simulink model "Power_Grid_Fault_Analysis_"  (R2019b)
settings: Solver=FixedStepAuto  StartTime=0.0  StopTime=0.2  RelTol=1e-3
InitFcn:
  | basekV = 23;
  | baseMVA = 100;
  | 
  | % base impedance
  | baseZ = (basekV)^2/baseMVA;
  | 
  | % nominal frequency
  | freq = 50;
libraries: powerlib x64, powerlib_meascontrol x17
(part 4 of 4)

== system Power_Grid_Fault_Analysis_/For Zone 2/If Action Subsystem1 ==
  Input : Inport
  Input1 : Inport  Port=2
  Input2 : Inport  Port=3
  Action Port : ActionPort  ActionPortLabel=elseif(u5 <= u1 & u1 <=u4 & u5 <= u3 & u3 <= u4 & u2 < u6)
  Out1 : Outport
  Out2 : Outport  Port=2
  Out3 : Outport  Port=3
  wires:
  Input/1 -> Out1/1
  Input1/1 -> Out2/1
  Input2/1 -> Out3/1

== system Power_Grid_Fault_Analysis_/For Zone 2/If Action Subsystem2 ==
  Input : Inport
  Input1 : Inport  Port=2
  Input2 : Inport  Port=3
  Action Port : ActionPort  ActionPortLabel=if(u5 <= u1 & u1 <=u4 & u5 <= u2 & u2 <=u4 & u3< u6)
  Out1 : Outport
  Out2 : Outport  Port=2
  Out3 : Outport  Port=3
  wires:
  Input/1 -> Out1/1
  Input1/1 -> Out2/1
  Input2/1 -> Out3/1

== system Power_Grid_Fault_Analysis_/For Zone 2/If Action Subsystem3 ==
  Input : Inport
  Input1 : Inport  Port=2
  Input2 : Inport  Port=3
  Action Port : ActionPort  ActionPortLabel=elseif(45 <= u3 & u3 <=u4 & u1 <= u7 & u2 <= u7)
  Out1 : Outport
  Out2 : Outport  Port=2
  Out3 : Outport  Port=3
  wires:
  Input/1 -> Out1/1
  Input1/1 -> Out2/1
  Input2/1 -> Out3/1

== system Power_Grid_Fault_Analysis_/For Zone 2/If Action Subsystem4 ==
  Input : Inport
  Input1 : Inport  Port=2
  Input2 : Inport  Port=3
  Action Port : ActionPort  ActionPortLabel="if(u1 >u5 & u2<u5 &  u3<u5)"
  Out1 : Outport
  Out2 : Outport  Port=2
  Out3 : Outport  Port=3
  wires:
  Input/1 -> Out1/1
  Input1/1 -> Out2/1
  Input2/1 -> Out3/1

== system Power_Grid_Fault_Analysis_/For Zone 2/If Action Subsystem5 ==
  Input : Inport
  Input1 : Inport  Port=2
  Input2 : Inport  Port=3
  Action Port : ActionPort  ActionPortLabel="elseif(u1 <u5 & u2>u5 &  u3<u5)"
  Out1 : Outport
  Out2 : Outport  Port=2
  Out3 : Outport  Port=3
  wires:
  Input/1 -> Out1/1
  Input1/1 -> Out2/1
  Input2/1 -> Out3/1

== system Power_Grid_Fault_Analysis_/For Zone 2/If Action Subsystem6 ==
  Input : Inport
  Input1 : Inport  Port=2
  Input2 : Inport  Port=3
  Action Port : ActionPort  ActionPortLabel="if(0<u1 & u1 < u4  &  u2 < u4 &  u3 <u4)"
  Out1 : Outport
  Out2 : Outport  Port=2
  Out3 : Outport  Port=3
  wires:
  Input/1 -> Out1/1
  Input1/1 -> Out2/1
  Input2/1 -> Out3/1

== system Power_Grid_Fault_Analysis_/For Zone 2/Subsystem1 ==
  In1 : Inport
  In2 : Inport  Port=2
  Display2 : Display
      settings: Decimation=2
  Divide4 : Product  Inputs=**  SaturateOnIntegerOverflow=on  RndMeth=Zero
  Output : Outport
  wires:
  Divide4/1 -> Display2/1, Output/1
  In1/1 -> Divide4/1
  In2/1 -> Divide4/2

== system Power_Grid_Fault_Analysis_/For Zone 2/Subsystem2 ==
  In1 : Inport
  In2 : Inport  Port=2
  Display2 : Display
      settings: Decimation=2
  Divide4 : Product  Inputs=**  SaturateOnIntegerOverflow=on  RndMeth=Zero
  Output : Outport
  wires:
  In2/1 -> Divide4/2
  In1/1 -> Divide4/1
  Divide4/1 -> Output/1, Display2/1

== system Power_Grid_Fault_Analysis_/For Zone 2/Subsystem3 ==
  In1 : Inport
  In2 : Inport  Port=2
  Display2 : Display
      settings: Decimation=2
  Divide4 : Product  Inputs=**  SaturateOnIntegerOverflow=on  RndMeth=Zero
  Output : Outport
  wires:
  In2/1 -> Divide4/2
  In1/1 -> Divide4/1
  Divide4/1 -> Output/1, Display2/1

== system Power_Grid_Fault_Analysis_/For Zone 2/Subsystem4 ==
  In1 : Inport
  In2 : Inport  Port=2
  Display2 : Display
      settings: Decimation=2
  Divide4 : Product  Inputs=**  SaturateOnIntegerOverflow=on  RndMeth=Zero
  Output : Outport
  wires:
  Divide4/1 -> Display2/1, Output/1
  In1/1 -> Divide4/1
  In2/1 -> Divide4/2

== system Power_Grid_Fault_Analysis_/For Zone 2/Subsystem5 ==
  In1 : Inport
  In2 : Inport  Port=2
  Display2 : Display
      settings: Decimation=2
  Divide4 : Product  Inputs=**  SaturateOnIntegerOverflow=on  RndMeth=Zero
  Output : Outport
  wires:
  In2/1 -> Divide4/2
  In1/1 -> Divide4/1
  Divide4/1 -> Output/1, Display2/1

== system Power_Grid_Fault_Analysis_/For Zone 2/Subsystem6 ==
  In1 : Inport
  In2 : Inport  Port=2
  Display2 : Display
      settings: Decimation=2
  Divide4 : Product  Inputs=**  SaturateOnIntegerOverflow=on  RndMeth=Zero
  Output : Outport
  wires:
  Divide4/1 -> Display2/1, Output/1
  In1/1 -> Divide4/1
  In2/1 -> Divide4/2

== system Power_Grid_Fault_Analysis_/For Zone 2/Subsystem7 ==
  In1 : Inport
  In2 : Inport  Port=2
  Display2 : Display
      settings: Decimation=2
  Divide4 : Product  Inputs=**  SaturateOnIntegerOverflow=on  RndMeth=Zero
  Output : Outport
  wires:
  In2/1 -> Divide4/2
  In1/1 -> Divide4/1
  Divide4/1 -> Output/1, Display2/1

== system Power_Grid_Fault_Analysis_/For Zone 3/If Action Subsystem ==
  Input : Inport
  Input1 : Inport  Port=2
  Input2 : Inport  Port=3
  Action Port : ActionPort  ActionPortLabel=if(u5 <= u2 & u2 <=u4 & u5 <= u3 & u3 <=u4 & u1 < u6)
  Out1 : Outport
  Out2 : Outport  Port=2
  Out3 : Outport  Port=3
  wires:
  Input/1 -> Out1/1
  Input1/1 -> Out2/1
  Input2/1 -> Out3/1

== system Power_Grid_Fault_Analysis_/For Zone 3/If Action Subsystem1 ==
  Input : Inport
  Input1 : Inport  Port=2
  Input2 : Inport  Port=3
  Action Port : ActionPort  ActionPortLabel=elseif(u5 <= u1 & u1 <=u4 & u5 <= u3 & u3 <= u4 & u2 < u6)
  Out1 : Outport
  Out2 : Outport  Port=2
  Out3 : Outport  Port=3
  wires:
  Input/1 -> Out1/1
  Input1/1 -> Out2/1
  Input2/1 -> Out3/1

== system Power_Grid_Fault_Analysis_/For Zone 3/If Action Subsystem2 ==
  Input : Inport
  Input1 : Inport  Port=2
  Input2 : Inport  Port=3
  Action Port : ActionPort  ActionPortLabel=if(u5 <= u1 & u1 <=u4 & u5 <= u2 & u2 <=u4 & u3< u6)
  Out1 : Outport
  Out2 : Outport  Port=2
  Out3 : Outport  Port=3
  wires:
  Input/1 -> Out1/1
  Input1/1 -> Out2/1
  Input2/1 -> Out3/1

== system Power_Grid_Fault_Analysis_/For Zone 3/If Action Subsystem3 ==
  Input : Inport
  Input1 : Inport  Port=2
  Input2 : Inport  Port=3
  Action Port : ActionPort  ActionPortLabel=elseif(15<= u3 & u3 <=u4 & u1 <= u7 & u2 <= u7)
  Out1 : Outport
  Out2 : Outport  Port=2
  Out3 : Outport  Port=3
  wires:
  Input/1 -> Out1/1
  Input1/1 -> Out2/1
  Input2/1 -> Out3/1

== system Power_Grid_Fault_Analysis_/For Zone 3/If Action Subsystem4 ==
  Input : Inport
  Input1 : Inport  Port=2
  Input2 : Inport  Port=3
  Action Port : ActionPort  ActionPortLabel="if(u1 >u5 & u2<u5 &  u3<u5)"
  Out1 : Outport
  Out2 : Outport  Port=2
  Out3 : Outport  Port=3
  wires:
  Input/1 -> Out1/1
  Input1/1 -> Out2/1
  Input2/1 -> Out3/1

== system Power_Grid_Fault_Analysis_/For Zone 3/If Action Subsystem5 ==
  Input : Inport
  Input1 : Inport  Port=2
  Input2 : Inport  Port=3
  Action Port : ActionPort  ActionPortLabel="elseif(u1 <u5 & u2>u5 &  u3<u5)"
  Out1 : Outport
  Out2 : Outport  Port=2
  Out3 : Outport  Port=3
  wires:
  Input/1 -> Out1/1
  Input1/1 -> Out2/1
  Input2/1 -> Out3/1

== system Power_Grid_Fault_Analysis_/For Zone 3/If Action Subsystem6 ==
  Input : Inport
  Input1 : Inport  Port=2
  Input2 : Inport  Port=3
  Action Port : ActionPort  ActionPortLabel="if(0<u1 & u1 < u4  &  u2 < u4 &  u3 <u4)"
  Out1 : Outport
  Out2 : Outport  Port=2
  Out3 : Outport  Port=3
  wires:
  Input/1 -> Out1/1
  Input1/1 -> Out2/1
  Input2/1 -> Out3/1

== system Power_Grid_Fault_Analysis_/For Zone 3/Subsystem1 ==
  In1 : Inport
  In2 : Inport  Port=2
  Display2 : Display
      settings: Decimation=2
  Divide4 : Product  Inputs=**  SaturateOnIntegerOverflow=on  RndMeth=Zero
  Output : Outport
  wires:
  Divide4/1 -> Display2/1, Output/1
  In1/1 -> Divide4/1
  In2/1 -> Divide4/2

== system Power_Grid_Fault_Analysis_/For Zone 3/Subsystem2 ==
  In1 : Inport
  In2 : Inport  Port=2
  Display2 : Display
      settings: Decimation=2
  Divide4 : Product  Inputs=**  SaturateOnIntegerOverflow=on  RndMeth=Zero
  Output : Outport
  wires:
  In2/1 -> Divide4/2
  In1/1 -> Divide4/1
  Divide4/1 -> Output/1, Display2/1

== system Power_Grid_Fault_Analysis_/For Zone 3/Subsystem3 ==
  In1 : Inport
  In2 : Inport  Port=2
  Display2 : Display
      settings: Decimation=2
  Divide4 : Product  Inputs=**  SaturateOnIntegerOverflow=on  RndMeth=Zero
  Output : Outport
  wires:
  In2/1 -> Divide4/2
  In1/1 -> Divide4/1
  Divide4/1 -> Output/1, Display2/1

== system Power_Grid_Fault_Analysis_/For Zone 3/Subsystem4 ==
  In1 : Inport
  In2 : Inport  Port=2
  Display2 : Display
      settings: Decimation=2
  Divide4 : Product  Inputs=**  SaturateOnIntegerOverflow=on  RndMeth=Zero
  Output : Outport
  wires:
  Divide4/1 -> Display2/1, Output/1
  In1/1 -> Divide4/1
  In2/1 -> Divide4/2

== system Power_Grid_Fault_Analysis_/For Zone 3/Subsystem5 ==
  In1 : Inport
  In2 : Inport  Port=2
  Display2 : Display
      settings: Decimation=2
  Divide4 : Product  Inputs=**  SaturateOnIntegerOverflow=on  RndMeth=Zero
  Output : Outport
  wires:
  In2/1 -> Divide4/2
  In1/1 -> Divide4/1
  Divide4/1 -> Output/1, Display2/1

== system Power_Grid_Fault_Analysis_/For Zone 3/Subsystem6 ==
  In1 : Inport
  In2 : Inport  Port=2
  Display2 : Display
      settings: Decimation=2
  Divide4 : Product  Inputs=**  SaturateOnIntegerOverflow=on  RndMeth=Zero
  Output : Outport
  wires:
  Divide4/1 -> Display2/1, Output/1
  In1/1 -> Divide4/1
  In2/1 -> Divide4/2

== system Power_Grid_Fault_Analysis_/For Zone 3/Subsystem7 ==
  In1 : Inport
  In2 : Inport  Port=2
  Display2 : Display
      settings: Decimation=2
  Divide4 : Product  Inputs=**  SaturateOnIntegerOverflow=on  RndMeth=Zero
  Output : Outport
  wires:
  In2/1 -> Divide4/2
  In1/1 -> Divide4/1
  Divide4/1 -> Output/1, Display2/1

== system Power_Grid_Fault_Analysis_/For Zone 4/If Action Subsystem ==
  Input : Inport
  Input1 : Inport  Port=2
  Input2 : Inport  Port=3
  Action Port : ActionPort  ActionPortLabel=if(u5 <= u2 & u2 <=u4 & u5 <= u3 & u3 <=u4 & u1 < u6)
  Out1 : Outport
  Out2 : Outport  Port=2
  Out3 : Outport  Port=3
  wires:
  Input/1 -> Out1/1
  Input1/1 -> Out2/1
  Input2/1 -> Out3/1

== system Power_Grid_Fault_Analysis_/For Zone 4/If Action Subsystem1 ==
  Input : Inport
  Input1 : Inport  Port=2
  Input2 : Inport  Port=3
  Action Port : ActionPort  ActionPortLabel=elseif(u5 <= u1 & u1 <=u4 & u5 <= u3 & u3 <= u4 & u2 < u6)
  Out1 : Outport
  Out2 : Outport  Port=2
  Out3 : Outport  Port=3
  wires:
  Input/1 -> Out1/1
  Input1/1 -> Out2/1
  Input2/1 -> Out3/1

== system Power_Grid_Fault_Analysis_/For Zone 4/If Action Subsystem2 ==
  Input : Inport
  Input1 : Inport  Port=2
  Input2 : Inport  Port=3
  Action Port : ActionPort  ActionPortLabel=if(u5 <= u1 & u1 <=u4 & u5 <= u2 & u2 <=u4 & u3< u6)
  Out1 : Outport
  Out2 : Outport  Port=2
  Out3 : Outport  Port=3
  wires:
  Input/1 -> Out1/1
  Input1/1 -> Out2/1
  Input2/1 -> Out3/1

== system Power_Grid_Fault_Analysis_/For Zone 4/If Action Subsystem3 ==
  Input : Inport
  Input1 : Inport  Port=2
  Input2 : Inport  Port=3
  Action Port : ActionPort  ActionPortLabel=elseif(120 <= u3 & u3 <=u4 & u1 <= u7 & u2 <= u7)
  Out1 : Outport
  Out2 : Outport  Port=2
  Out3 : Outport  Port=3
  wires:
  Input/1 -> Out1/1
  Input1/1 -> Out2/1
  Input2/1 -> Out3/1

== system Power_Grid_Fault_Analysis_/For Zone 4/If Action Subsystem4 ==
  Input : Inport
  Input1 : Inport  Port=2
  Input2 : Inport  Port=3
  Action Port : ActionPort  ActionPortLabel="if(u1 >u5 & u2<u5 &  u3<u5)"
  Out1 : Outport
  Out2 : Outport  Port=2
  Out3 : Outport  Port=3
  wires:
  Input/1 -> Out1/1
  Input1/1 -> Out2/1
  Input2/1 -> Out3/1

== system Power_Grid_Fault_Analysis_/For Zone 4/If Action Subsystem5 ==
  Input : Inport
  Input1 : Inport  Port=2
  Input2 : Inport  Port=3
  Action Port : ActionPort  ActionPortLabel="elseif(u1 <u5 & u2>u5 &  u3<u5)"
  Out1 : Outport
  Out2 : Outport  Port=2
  Out3 : Outport  Port=3
  wires:
  Input/1 -> Out1/1
  Input1/1 -> Out2/1
  Input2/1 -> Out3/1

== system Power_Grid_Fault_Analysis_/For Zone 4/If Action Subsystem6 ==
  Input : Inport
  Input1 : Inport  Port=2
  Input2 : Inport  Port=3
  Action Port : ActionPort  ActionPortLabel="if(0<u1 & u1 < u4  &  u2 < u4 &  u3 <u4)"
  Out1 : Outport
  Out2 : Outport  Port=2
  Out3 : Outport  Port=3
  wires:
  Input/1 -> Out1/1
  Input1/1 -> Out2/1
  Input2/1 -> Out3/1

== system Power_Grid_Fault_Analysis_/For Zone 4/Subsystem1 ==
  In1 : Inport
  In2 : Inport  Port=2
  Display2 : Display
      settings: Decimation=2
  Divide4 : Product  Inputs=**  SaturateOnIntegerOverflow=on  RndMeth=Zero
  Output : Outport
  wires:
  Divide4/1 -> Display2/1, Output/1
  In1/1 -> Divide4/1
  In2/1 -> Divide4/2

== system Power_Grid_Fault_Analysis_/For Zone 4/Subsystem2 ==
  In1 : Inport
  In2 : Inport  Port=2
  Display2 : Display
      settings: Decimation=2
  Divide4 : Product  Inputs=**  SaturateOnIntegerOverflow=on  RndMeth=Zero
  Output : Outport
  wires:
  In2/1 -> Divide4/2
  In1/1 -> Divide4/1
  Divide4/1 -> Output/1, Display2/1

== system Power_Grid_Fault_Analysis_/For Zone 4/Subsystem3 ==
  In1 : Inport
  In2 : Inport  Port=2
  Display2 : Display
      settings: Decimation=2
  Divide4 : Product  Inputs=**  SaturateOnIntegerOverflow=on  RndMeth=Zero
  Output : Outport
  wires:
  In2/1 -> Divide4/2
  In1/1 -> Divide4/1
  Divide4/1 -> Output/1, Display2/1

== system Power_Grid_Fault_Analysis_/For Zone 4/Subsystem4 ==
  In1 : Inport
  In2 : Inport  Port=2
  Display2 : Display
      settings: Decimation=2
  Divide4 : Product  Inputs=**  SaturateOnIntegerOverflow=on  RndMeth=Zero
  Output : Outport
  wires:
  Divide4/1 -> Display2/1, Output/1
  In1/1 -> Divide4/1
  In2/1 -> Divide4/2

== system Power_Grid_Fault_Analysis_/For Zone 4/Subsystem5 ==
  In1 : Inport
  In2 : Inport  Port=2
  Display2 : Display
      settings: Decimation=2
  Divide4 : Product  Inputs=**  SaturateOnIntegerOverflow=on  RndMeth=Zero
  Output : Outport
  wires:
  In2/1 -> Divide4/2
  In1/1 -> Divide4/1
  Divide4/1 -> Output/1, Display2/1

== system Power_Grid_Fault_Analysis_/For Zone 4/Subsystem6 ==
  In1 : Inport
  In2 : Inport  Port=2
  Display2 : Display
      settings: Decimation=2
  Divide4 : Product  Inputs=**  SaturateOnIntegerOverflow=on  RndMeth=Zero
  Output : Outport
  wires:
  Divide4/1 -> Display2/1, Output/1
  In1/1 -> Divide4/1
  In2/1 -> Divide4/2

== system Power_Grid_Fault_Analysis_/For Zone 4/Subsystem7 ==
  In1 : Inport
  In2 : Inport  Port=2
  Display2 : Display
      settings: Decimation=2
  Divide4 : Product  Inputs=**  SaturateOnIntegerOverflow=on  RndMeth=Zero
  Output : Outport
  wires:
  In2/1 -> Divide4/2
  In1/1 -> Divide4/1
  Divide4/1 -> Output/1, Display2/1

== system Power_Grid_Fault_Analysis_/For Zone 5/If Action Subsystem ==
  Input : Inport
  Input1 : Inport  Port=2
  Input2 : Inport  Port=3
  Action Port : ActionPort  ActionPortLabel=if(u5 <= u2 & u2 <=u4 & u5 <= u3 & u3 <=u4 & u1 < u6)
  Out1 : Outport
  Out2 : Outport  Port=2
  Out3 : Outport  Port=3
  wires:
  Input/1 -> Out1/1
  Input1/1 -> Out2/1
  Input2/1 -> Out3/1

== system Power_Grid_Fault_Analysis_/For Zone 5/If Action Subsystem1 ==
  Input : Inport
  Input1 : Inport  Port=2
  Input2 : Inport  Port=3
  Action Port : ActionPort  ActionPortLabel=elseif(u5 <= u1 & u1 <=u4 & u5 <= u3 & u3 <= u4 & u2 < u6)
  Out1 : Outport
  Out2 : Outport  Port=2
  Out3 : Outport  Port=3
  wires:
  Input/1 -> Out1/1
  Input1/1 -> Out2/1
  Input2/1 -> Out3/1

== system Power_Grid_Fault_Analysis_/For Zone 5/If Action Subsystem2 ==
  Input : Inport
  Input1 : Inport  Port=2
  Input2 : Inport  Port=3
  Action Port : ActionPort  ActionPortLabel=if(u5 <= u1 & u1 <=u4 & u5 <= u2 & u2 <=u4 & u3< u6)
  Out1 : Outport
  Out2 : Outport  Port=2
  Out3 : Outport  Port=3
  wires:
  Input/1 -> Out1/1
  Input1/1 -> Out2/1
  Input2/1 -> Out3/1

== system Power_Grid_Fault_Analysis_/For Zone 5/If Action Subsystem3 ==
  Input : Inport
  Input1 : Inport  Port=2
  Input2 : Inport  Port=3
  Action Port : ActionPort  ActionPortLabel=elseif(50 <= u3 & u3 <=u4 & u1 <= u7 & u2 <= u7)
  Out1 : Outport
  Out2 : Outport  Port=2
  Out3 : Outport  Port=3
  wires:
  Input/1 -> Out1/1
  Input1/1 -> Out2/1
  Input2/1 -> Out3/1

== system Power_Grid_Fault_Analysis_/For Zone 5/If Action Subsystem4 ==
  Input : Inport
  Input1 : Inport  Port=2
  Input2 : Inport  Port=3
  Action Port : ActionPort  ActionPortLabel="if(u1 >u5 & u2<u5 &  u3<u5)"
  Out1 : Outport
  Out2 : Outport  Port=2
  Out3 : Outport  Port=3
  wires:
  Input/1 -> Out1/1
  Input1/1 -> Out2/1
  Input2/1 -> Out3/1

== system Power_Grid_Fault_Analysis_/For Zone 5/If Action Subsystem5 ==
  Input : Inport
  Input1 : Inport  Port=2
  Input2 : Inport  Port=3
  Action Port : ActionPort  ActionPortLabel="elseif(u1 <u5 & u2>u5 &  u3<u5)"
  Out1 : Outport
  Out2 : Outport  Port=2
  Out3 : Outport  Port=3
  wires:
  Input/1 -> Out1/1
  Input1/1 -> Out2/1
  Input2/1 -> Out3/1

== system Power_Grid_Fault_Analysis_/For Zone 5/If Action Subsystem6 ==
  Input : Inport
  Input1 : Inport  Port=2
  Input2 : Inport  Port=3
  Action Port : ActionPort  ActionPortLabel="if(0<u1 & u1 < u4  &  u2 < u4 &  u3 <u4)"
  Out1 : Outport
  Out2 : Outport  Port=2
  Out3 : Outport  Port=3
  wires:
  Input/1 -> Out1/1
  Input1/1 -> Out2/1
  Input2/1 -> Out3/1

== system Power_Grid_Fault_Analysis_/For Zone 5/Subsystem1 ==
  In1 : Inport
  In2 : Inport  Port=2
  Display2 : Display
      settings: Decimation=2
  Divide4 : Product  Inputs=**  SaturateOnIntegerOverflow=on  RndMeth=Zero
  Output : Outport
  wires:
  Divide4/1 -> Display2/1, Output/1
  In1/1 -> Divide4/1
  In2/1 -> Divide4/2

== system Power_Grid_Fault_Analysis_/For Zone 5/Subsystem2 ==
  In1 : Inport
  In2 : Inport  Port=2
  Display2 : Display
      settings: Decimation=2
  Divide4 : Product  Inputs=**  SaturateOnIntegerOverflow=on  RndMeth=Zero
  Output : Outport
  wires:
  In2/1 -> Divide4/2
  In1/1 -> Divide4/1
  Divide4/1 -> Output/1, Display2/1

== system Power_Grid_Fault_Analysis_/For Zone 5/Subsystem3 ==
  In1 : Inport
  In2 : Inport  Port=2
  Display2 : Display
      settings: Decimation=2
  Divide4 : Product  Inputs=**  SaturateOnIntegerOverflow=on  RndMeth=Zero
  Output : Outport
  wires:
  In2/1 -> Divide4/2
  In1/1 -> Divide4/1
  Divide4/1 -> Output/1, Display2/1

== system Power_Grid_Fault_Analysis_/For Zone 5/Subsystem4 ==
  In1 : Inport
  In2 : Inport  Port=2
  Display2 : Display
      settings: Decimation=2
  Divide4 : Product  Inputs=**  SaturateOnIntegerOverflow=on  RndMeth=Zero
  Output : Outport
  wires:
  Divide4/1 -> Display2/1, Output/1
  In1/1 -> Divide4/1
  In2/1 -> Divide4/2

== system Power_Grid_Fault_Analysis_/For Zone 5/Subsystem5 ==
  In1 : Inport
  In2 : Inport  Port=2
  Display2 : Display
      settings: Decimation=2
  Divide4 : Product  Inputs=**  SaturateOnIntegerOverflow=on  RndMeth=Zero
  Output : Outport
  wires:
  In2/1 -> Divide4/2
  In1/1 -> Divide4/1
  Divide4/1 -> Output/1, Display2/1

== system Power_Grid_Fault_Analysis_/For Zone 5/Subsystem6 ==
  In1 : Inport
  In2 : Inport  Port=2
  Display2 : Display
      settings: Decimation=2
  Divide4 : Product  Inputs=**  SaturateOnIntegerOverflow=on  RndMeth=Zero
  Output : Outport
  wires:
  Divide4/1 -> Display2/1, Output/1
  In1/1 -> Divide4/1
  In2/1 -> Divide4/2

== system Power_Grid_Fault_Analysis_/For Zone 5/Subsystem7 ==
  In1 : Inport
  In2 : Inport  Port=2
  Display2 : Display
      settings: Decimation=2
  Divide4 : Product  Inputs=**  SaturateOnIntegerOverflow=on  RndMeth=Zero
  Output : Outport
  wires:
  In2/1 -> Divide4/2
  In1/1 -> Divide4/1
  Divide4/1 -> Output/1, Display2/1

== system Power_Grid_Fault_Analysis_/Relay /AC Time Overcurrent Relay2 ==
  I : Inport
  Clock : Clock
  Irms : powerlib_meascontrol/Measurements/RMS  TrueRMS=on  Freq=Freq  RMSInit=RMSInit  Ts=0
      settings: SourceProductName=Simscape Electrical
  Relational Operator : RelationalOperator  Operator=<=  OutDataTypeStr=boolean  RndMeth=Nearest
  Time Relay Function : MATLAB Function  TreatAsAtomicUnit=on
  C.B : Outport
  OT : Outport  Port=2
  wires:
  Clock/1 -> Relational Operator/1, Time Relay Function/1(clk)
  Irms/1 -> Time Relay Function/2(Irms)
  Time Relay Function/1(TT) -> Relational Operator/2
  Time Relay Function/2(OT) -> OT/1
  Relational Operator/1 -> C.B/1
  I/1 -> Irms/1

== system Power_Grid_Fault_Analysis_/Relay /Output1 ==
  Signal : Inport
  Demux : Demux  Outputs=3
  Scope : Scope  NumInputPorts=3
  wires:
  Demux/3 -> Scope/3
  Demux/1 -> Scope/1
  Demux/2 -> Scope/2
  Signal/1 -> Demux/1

== system Power_Grid_Fault_Analysis_/Relay /Subsystem ==
  In1 : Inport
  Constant : Constant  Value=5
  Data Type Conversion : DataTypeConversion  OutDataTypeStr=boolean
  Display1 : Display
  NOT : Logic  Operator=NOT  IconShape=distinctive  AllPortsSameDT=off  OutDataTypeStr=boolean
  Sum : Sum  Inputs=|+-
  To Workspace : ToWorkspace  VariableName=G_F_1  SaveFormat=Timeseries  SampleTime=-1
  wires:
  Data Type Conversion/1 -> NOT/1
  Constant/1 -> Sum/2
  Sum/1 -> Data Type Conversion/1
  In1/1 -> To Workspace/1, Sum/1
  NOT/1 -> Display1/1

== system Power_Grid_Fault_Analysis_/Relay 1/AC Time Overcurrent Relay2 ==
  I : Inport
  Clock : Clock
  Irms : powerlib_meascontrol/Measurements/RMS  TrueRMS=on  Freq=Freq  RMSInit=RMSInit  Ts=0
      settings: SourceProductName=Simscape Electrical
  Relational Operator : RelationalOperator  Operator=<=  OutDataTypeStr=boolean  RndMeth=Nearest
  Time Relay Function : MATLAB Function  TreatAsAtomicUnit=on
  C.B : Outport
  OT : Outport  Port=2
  wires:
  Clock/1 -> Relational Operator/1, Time Relay Function/1(clk)
  Irms/1 -> Time Relay Function/2(Irms)
  Time Relay Function/1(TT) -> Relational Operator/2
  Time Relay Function/2(OT) -> OT/1
  Relational Operator/1 -> C.B/1
  I/1 -> Irms/1

== system Power_Grid_Fault_Analysis_/Relay 1/Output1 ==
  Signal : Inport
  Demux : Demux  Outputs=3
  Scope : Scope  NumInputPorts=3
  wires:
  Demux/3 -> Scope/3
  Demux/1 -> Scope/1
  Demux/2 -> Scope/2
  Signal/1 -> Demux/1

== system Power_Grid_Fault_Analysis_/Relay 1/Subsystem ==
  In1 : Inport
  Constant : Constant  Value=5
  Data Type Conversion : DataTypeConversion  OutDataTypeStr=boolean
  Display1 : Display
  NOT : Logic  Operator=NOT  IconShape=distinctive  AllPortsSameDT=off  OutDataTypeStr=boolean
  Sum : Sum  Inputs=|+-
  To Workspace : ToWorkspace  VariableName=G_F_R_1  SaveFormat=Timeseries  SampleTime=-1
  wires:
  Data Type Conversion/1 -> NOT/1
  Constant/1 -> Sum/2
  Sum/1 -> Data Type Conversion/1
  In1/1 -> To Workspace/1, Sum/1
  NOT/1 -> Display1/1

== system Power_Grid_Fault_Analysis_/Relay 2/AC Time Overcurrent Relay2 ==
  I : Inport
  Clock : Clock
  Irms : powerlib_meascontrol/Measurements/RMS  TrueRMS=on  Freq=Freq  RMSInit=RMSInit  Ts=0
      settings: SourceProductName=Simscape Electrical
  Relational Operator : RelationalOperator  Operator=<=  OutDataTypeStr=boolean  RndMeth=Nearest
  Time Relay Function : MATLAB Function  TreatAsAtomicUnit=on
  C.B : Outport
  OT : Outport  Port=2
  wires:
  Clock/1 -> Relational Operator/1, Time Relay Function/1(clk)
  Irms/1 -> Time Relay Function/2(Irms)
  Time Relay Function/1(TT) -> Relational Operator/2
  Time Relay Function/2(OT) -> OT/1
  Relational Operator/1 -> C.B/1
  I/1 -> Irms/1

== system Power_Grid_Fault_Analysis_/Relay 2/Output1 ==
  Signal : Inport
  Demux : Demux  Outputs=3
  Scope : Scope  NumInputPorts=3
  wires:
  Demux/3 -> Scope/3
  Demux/1 -> Scope/1
  Demux/2 -> Scope/2
  Signal/1 -> Demux/1

== system Power_Grid_Fault_Analysis_/Relay 2/Subsystem ==
  In1 : Inport
  Constant : Constant  Value=5
  Data Type Conversion : DataTypeConversion  OutDataTypeStr=boolean
  Display1 : Display
  NOT : Logic  Operator=NOT  IconShape=distinctive  AllPortsSameDT=off  OutDataTypeStr=boolean
  Sum : Sum  Inputs=|+-
  To Workspace : ToWorkspace  VariableName=G_F_R_2  SaveFormat=Timeseries  SampleTime=-1
  wires:
  Data Type Conversion/1 -> NOT/1
  Constant/1 -> Sum/2
  Sum/1 -> Data Type Conversion/1
  In1/1 -> To Workspace/1, Sum/1
  NOT/1 -> Display1/1

== system Power_Grid_Fault_Analysis_/Relay 3/AC Time Overcurrent Relay2 ==
  I : Inport
  Clock : Clock
  Irms : powerlib_meascontrol/Measurements/RMS  TrueRMS=on  Freq=Freq  RMSInit=RMSInit  Ts=0
      settings: SourceProductName=Simscape Electrical
  Relational Operator : RelationalOperator  Operator=<=  OutDataTypeStr=boolean  RndMeth=Nearest
  Time Relay Function : MATLAB Function  TreatAsAtomicUnit=on
  C.B : Outport
  OT : Outport  Port=2
  wires:
  Clock/1 -> Relational Operator/1, Time Relay Function/1(clk)
  Irms/1 -> Time Relay Function/2(Irms)
  Time Relay Function/1(TT) -> Relational Operator/2
  Time Relay Function/2(OT) -> OT/1
  Relational Operator/1 -> C.B/1
  I/1 -> Irms/1

== system Power_Grid_Fault_Analysis_/Relay 3/Output1 ==
  Signal : Inport
  Demux : Demux  Outputs=3
  Scope : Scope  NumInputPorts=3
  wires:
  Demux/3 -> Scope/3
  Demux/1 -> Scope/1
  Demux/2 -> Scope/2
  Signal/1 -> Demux/1

== system Power_Grid_Fault_Analysis_/Relay 3/Subsystem ==
  In1 : Inport
  Constant : Constant  Value=5
  Data Type Conversion : DataTypeConversion  OutDataTypeStr=boolean
  Display1 : Display
  NOT : Logic  Operator=NOT  IconShape=distinctive  AllPortsSameDT=off  OutDataTypeStr=boolean
  Sum : Sum  Inputs=|+-
  To Workspace : ToWorkspace  VariableName=G_F_R_3  SaveFormat=Timeseries  SampleTime=-1
  wires:
  Data Type Conversion/1 -> NOT/1
  Constant/1 -> Sum/2
  Sum/1 -> Data Type Conversion/1
  In1/1 -> To Workspace/1, Sum/1
  NOT/1 -> Display1/1

== system Power_Grid_Fault_Analysis_/Relay 4/AC Time Overcurrent Relay2 ==
  I : Inport
  Clock : Clock
  Irms : powerlib_meascontrol/Measurements/RMS  TrueRMS=on  Freq=Freq  RMSInit=RMSInit  Ts=0
      settings: SourceProductName=Simscape Electrical
  Relational Operator : RelationalOperator  Operator=<=  OutDataTypeStr=boolean  RndMeth=Nearest
  Time Relay Function : MATLAB Function  TreatAsAtomicUnit=on
  C.B : Outport
  OT : Outport  Port=2
  wires:
  Clock/1 -> Relational Operator/1, Time Relay Function/1(clk)
  Irms/1 -> Time Relay Function/2(Irms)
  Time Relay Function/1(TT) -> Relational Operator/2
  Time Relay Function/2(OT) -> OT/1
  Relational Operator/1 -> C.B/1
  I/1 -> Irms/1

== system Power_Grid_Fault_Analysis_/Relay 4/Output1 ==
  Signal : Inport
  Demux : Demux  Outputs=3
  Scope : Scope  NumInputPorts=3
  wires:
  Demux/3 -> Scope/3
  Demux/1 -> Scope/1
  Demux/2 -> Scope/2
  Signal/1 -> Demux/1

== system Power_Grid_Fault_Analysis_/Relay 4/Subsystem ==
  In1 : Inport
  Constant : Constant  Value=5
  Data Type Conversion : DataTypeConversion  OutDataTypeStr=boolean
  Display1 : Display
  NOT : Logic  Operator=NOT  IconShape=distinctive  AllPortsSameDT=off  OutDataTypeStr=boolean
  Sum : Sum  Inputs=|+-
  To Workspace : ToWorkspace  VariableName=G_F_R_4  SaveFormat=Timeseries  SampleTime=-1
  wires:
  Data Type Conversion/1 -> NOT/1
  Constant/1 -> Sum/2
  Sum/1 -> Data Type Conversion/1
  In1/1 -> To Workspace/1, Sum/1
  NOT/1 -> Display1/1

== matlab function Power_Grid_Fault_Analysis_/Relay 1/AC Time Overcurrent Relay2/Time Relay Function ==
  settings: updateMethod=DISCRETE
  data: TT output; clk input; Irms input; CTpri parameter; CTsec parameter; PS parameter; OT output; TMS parameter; k parameter; alpha parameter; B parameter; TDS parameter
function [TT, OT] = fcn(clk,Irms,CTpri,CTsec,PS,TMS,k,alpha,B,TDS)

persistent RelayState TripTime OperatingTime PickupTime

if isempty(RelayState)
    RelayState = 0;
    TripTime = inf;
    OperatingTime = inf;
    PickupTime = 0;
end

CT = max(Irms/(CTpri/CTsec));
Pickup = (PS*0.25)*CTsec;

if (RelayState == 0)&&(CT > Pickup)
    PickupTime = clk;
    RelayState = 1;
end

if (RelayState == 1)&&(clk>(PickupTime+0.02)) % Wait for 20ms fault current rise time
    if k == 0
        OperatingTime = TDS;
    else
        PMS = CT/Pickup;                          % Calculate Plug Multiplier Setting
        OperatingTime = ((k/((PMS^alpha)-1))+B)*(TMS*0.05); % Determine Definite Inverse Minimum Time
    end
    TripTime = PickupTime + OperatingTime;
    RelayState = 2;
end

TT = TripTime;
OT = OperatingTime;

== matlab function Power_Grid_Fault_Analysis_/Relay 2/AC Time Overcurrent Relay2/Time Relay Function ==
  settings: updateMethod=DISCRETE
  data: TT output; clk input; Irms input; CTpri parameter; CTsec parameter; PS parameter; OT output; TMS parameter; k parameter; alpha parameter; B parameter; TDS parameter
function [TT, OT] = fcn(clk,Irms,CTpri,CTsec,PS,TMS,k,alpha,B,TDS)

persistent RelayState TripTime OperatingTime PickupTime

if isempty(RelayState)
    RelayState = 0;
    TripTime = inf;
    OperatingTime = inf;
    PickupTime = 0;
end

CT = max(Irms/(CTpri/CTsec));
Pickup = (PS*0.25)*CTsec;

if (RelayState == 0)&&(CT > Pickup)
    PickupTime = clk;
    RelayState = 1;
end

if (RelayState == 1)&&(clk>(PickupTime+0.02)) % Wait for 20ms fault current rise time
    if k == 0
        OperatingTime = TDS;
    else
        PMS = CT/Pickup;                          % Calculate Plug Multiplier Setting
        OperatingTime = ((k/((PMS^alpha)-1))+B)*(TMS*0.05); % Determine Definite Inverse Minimum Time
    end
    TripTime = PickupTime + OperatingTime;
    RelayState = 2;
end

TT = TripTime;
OT = OperatingTime;

== matlab function Power_Grid_Fault_Analysis_/Relay /AC Time Overcurrent Relay2/Time Relay Function ==
  settings: updateMethod=DISCRETE
  data: TT output; clk input; Irms input; CTpri parameter; CTsec parameter; PS parameter; OT output; TMS parameter; k parameter; alpha parameter; B parameter; TDS parameter
function [TT, OT] = fcn(clk,Irms,CTpri,CTsec,PS,TMS,k,alpha,B,TDS)

persistent RelayState TripTime OperatingTime PickupTime

if isempty(RelayState)
    RelayState = 0;
    TripTime = inf;
    OperatingTime = inf;
    PickupTime = 0;
end

CT = max(Irms/(CTpri/CTsec));
Pickup = (PS*0.25)*CTsec;

if (RelayState == 0)&&(CT > Pickup)
    PickupTime = clk;
    RelayState = 1;
end

if (RelayState == 1)&&(clk>(PickupTime+0.02)) % Wait for 20ms fault current rise time
    if k == 0
        OperatingTime = TDS;
    else
        PMS = CT/Pickup;                          % Calculate Plug Multiplier Setting
        OperatingTime = ((k/((PMS^alpha)-1))+B)*(TMS*0.05); % Determine Definite Inverse Minimum Time
    end
    TripTime = PickupTime + OperatingTime;
    RelayState = 2;
end

TT = TripTime;
OT = OperatingTime;

== matlab function Power_Grid_Fault_Analysis_/Relay 3/AC Time Overcurrent Relay2/Time Relay Function ==
  settings: updateMethod=DISCRETE
  data: TT output; clk input; Irms input; CTpri parameter; CTsec parameter; PS parameter; OT output; TMS parameter; k parameter; alpha parameter; B parameter; TDS parameter
function [TT, OT] = fcn(clk,Irms,CTpri,CTsec,PS,TMS,k,alpha,B,TDS)

persistent RelayState TripTime OperatingTime PickupTime

if isempty(RelayState)
    RelayState = 0;
    TripTime = inf;
    OperatingTime = inf;
    PickupTime = 0;
end

CT = max(Irms/(CTpri/CTsec));
Pickup = (PS*0.25)*CTsec;

if (RelayState == 0)&&(CT > Pickup)
    PickupTime = clk;
    RelayState = 1;
end

if (RelayState == 1)&&(clk>(PickupTime+0.02)) % Wait for 20ms fault current rise time
    if k == 0
        OperatingTime = TDS;
    else
        PMS = CT/Pickup;                          % Calculate Plug Multiplier Setting
        OperatingTime = ((k/((PMS^alpha)-1))+B)*(TMS*0.05); % Determine Definite Inverse Minimum Time
    end
    TripTime = PickupTime + OperatingTime;
    RelayState = 2;
end

TT = TripTime;
OT = OperatingTime;

== matlab function Power_Grid_Fault_Analysis_/Relay 4/AC Time Overcurrent Relay2/Time Relay Function ==
  settings: updateMethod=DISCRETE
  data: TT output; clk input; Irms input; CTpri parameter; CTsec parameter; PS parameter; OT output; TMS parameter; k parameter; alpha parameter; B parameter; TDS parameter
function [TT, OT] = fcn(clk,Irms,CTpri,CTsec,PS,TMS,k,alpha,B,TDS)

persistent RelayState TripTime OperatingTime PickupTime

if isempty(RelayState)
    RelayState = 0;
    TripTime = inf;
    OperatingTime = inf;
    PickupTime = 0;
end

CT = max(Irms/(CTpri/CTsec));
Pickup = (PS*0.25)*CTsec;

if (RelayState == 0)&&(CT > Pickup)
    PickupTime = clk;
    RelayState = 1;
end

if (RelayState == 1)&&(clk>(PickupTime+0.02)) % Wait for 20ms fault current rise time
    if k == 0
        OperatingTime = TDS;
    else
        PMS = CT/Pickup;                          % Calculate Plug Multiplier Setting
        OperatingTime = ((k/((PMS^alpha)-1))+B)*(TMS*0.05); % Determine Definite Inverse Minimum Time
    end
    TripTime = PickupTime + OperatingTime;
    RelayState = 2;
end

TT = TripTime;
OT = OperatingTime;
